simulink model "Exo_Origianl"  (R2023b)
settings: Solver=ode5  StartTime=0.0  StopTime=inf  FixedStep=dt  RelTol=1e-3  EnableMultiTasking=on
values from neighbouring files (symbols this model uses):
  A_0_a = 4.011    [Operator.m]
  A_0_h = 40.69    [Operator.m]
  A_0_k = 25.7    [Operator.m]
  A_1_a = 5.292    [Operator.m]
  A_1_h = 23.22    [Operator.m]
  A_1_k = -3.827    [Operator.m]
  A_2_a = -8.582    [Operator.m]
  A_2_h = -4.487    [Operator.m]
  A_2_k = -8.543    [Operator.m]
  A_3_a = -0.4755    [Operator.m]
  A_3_h = 0.3995    [Operator.m]
  A_3_k = 1.913    [Operator.m]
  A_4_a = 1.688    [Operator.m]
  A_4_k = 1.087    [Operator.m]
  A_5_a = -0.03504    [Operator.m]
  A_5_k = 2.054    [Operator.m]
  A_6_a = 1.298    [Operator.m]
  A_6_k = -0.3061    [Operator.m]
  amplitude = 0.8    [Operator.m]
  ankleStrategyInterval = 1.5    [Operator.m]
  B_1_a = 3.613    [Operator.m]
  B_1_h = -8.65    [Operator.m]
  B_1_k = -19.28    [Operator.m]
  B_2_a = -5.954    [Operator.m]
  B_2_h = 3.338    [Operator.m]
  B_2_k = 17.93    [Operator.m]
  B_3_a = 5.918    [Operator.m]
  B_3_h = 1.389    [Operator.m]
  B_3_k = 3.772    [Operator.m]
  B_4_a = -2.118    [Operator.m]
  B_4_k = 1.504    [Operator.m]
  B_5_a = 1.023    [Operator.m]
  B_5_k = 0.5838    [Operator.m]
  B_6_a = -0.7245    [Operator.m]
  B_6_k = -0.8958    [Operator.m]
  DCM_filter = 1 - dt/(dt+RC)    (= 0.926612305411)    [Operator.m]
  dt = 0.01    [Operator.m]
  frequency = 1.2    [Operator.m]
  gamma = fzero(eqn, 0.1)    [Operator.m]
  hipOffset = -17    [Operator.m]
  K_high = 0.5    [Operator.m]
  K_low = 0.5    [Operator.m]
  KD = 0.39    [Operator.m]
  Kp = 10    [Operator.m]
  l3 = userHeight*0.232    (= 15.776)    [Operator.m]
  l4 = userHeight*0.247    (= 16.796)    [Operator.m]
  l_c2 = ((0.29*34.66+0.63*6.07)/(6.07+34.66))/(0.52+0.19)*l2    (= 15.0425832454)    [Operator.m]
  l_c3 = 0.17/0.40*l3    (= 6.7048)    [Operator.m]
  l_c4 = ((0.19*3.52+0.43*1.05)/(3.52+1.05))/0.43*l4    (= 9.57536959951)    [Operator.m]
  l_foot = 11.25    [Operator.m]
  m2 = m2 + 2.2048*7.591    (= 119.8566368)    [Operator.m]
  m3 = m3 + 2.2048*1.715    (= 19.781232)    [Operator.m]
  m4 = userWeight*(0.0459+0.0169)    (= 10.048)    [Operator.m]
  m_Exo = 2.2048*1.647    (= 3.6313056)    [Operator.m]
  m_f = userWeight*0.0169    (= 2.704)    [Operator.m]
  maxTorque = 35    [Operator.m]
  P_t_ZMP_gain_Ankle = 0    [Operator.m]
  P_t_ZMP_gain_Hip = 0    [Operator.m]
  Phase_Left = 2+pi    (= 5.14159265359)    [Operator.m]
  Phase_Right = 2    [Operator.m]
  ramp = 2    [Operator.m]
  Strategy_filter = DCM_filter    (= 0.926612305411)    [Operator.m]
  strategySaturation = 10    [Operator.m]
  userHeight = 68    [Operator.m]
  userWeight = 160    [Operator.m]
undefined symbols (not defined in the file or in its folder): CAN_Device, DCMErrorPenalty, PEAK, Phase_Left_Knee_0, System, totalPowerPenalty
libraries: sldrtlib x35, simulink x16, rllib x1
(part 2 of 4)

== system Exo_Origianl/Subsystem1 ==
  In1 : Inport
  In2 : Inport  Port=2
  Trigger : TriggerPort  VariantControl=(inherit)  PortDimensions=1
  Constant{1..6} (6 alike) : Constant  Value=3
  Packet Output : sldrtlib/Packet Output  SampleTime=-1  MaxMissedTicks=100  ShowMissedTicks=off  YieldWhenWaiting=off  DrvName=PEAK-System/CAN_Device  DrvAddress=81  DrvOptions=[0 0 0 0 1000 0 0 1 5 2 1 3 1]  PacketSize=8  DataTypes={'uint8','uint8','uint8','uint8','uint8','uint8','uint8','uint8'}  ShowReady=off  ShowError=off  PacketID=2048e0 + (81)  ByteOrder=2  InitialValue=[]  FinalValue=[]
      settings: AttributesFormatString=PEAK-System\nCAN Device [81]
  wires:
  In2/1 -> Packet Output/2
  In1/1 -> Packet Output/1
  Constant1/1 -> Packet Output/7
  Constant6/1 -> Packet Output/8
  Constant2/1 -> Packet Output/3
  Constant3/1 -> Packet Output/4
  Constant4/1 -> Packet Output/5
  Constant5/1 -> Packet Output/6

== system Exo_Origianl/Subsystem10 ==
  In1 : Inport
  Trigger : TriggerPort  TriggerType=either  VariantControl=(inherit)  PortDimensions=1
  Constant{1..7} (7 alike) : Constant
  Packet Output : sldrtlib/Packet Output  SampleTime=-1  MaxMissedTicks=100  ShowMissedTicks=off  YieldWhenWaiting=off  DrvName=PEAK-System/CAN_Device  DrvAddress=81  DrvOptions=[0 0 0 0 1000 0 0 1 5 2 1 3 1]  PacketSize=8  DataTypes={'uint8','uint8','uint8','uint8','uint8','uint8','uint8','uint8'}  ShowReady=off  ShowError=off  PacketID=2048e0 + (85)  ByteOrder=2  InitialValue=[]  FinalValue=[]
      settings: AttributesFormatString=PEAK-System\nCAN Device [81]
  wires:
  Constant7/1 -> Packet Output/2
  In1/1 -> Packet Output/1
  Constant3/1 -> Packet Output/4
  Constant1/1 -> Packet Output/7
  Constant6/1 -> Packet Output/8
  Constant4/1 -> Packet Output/5
  Constant2/1 -> Packet Output/3
  Constant5/1 -> Packet Output/6

== system Exo_Origianl/Subsystem11 ==
  In1 : Inport
  In2 : Inport  Port=2
  Trigger : TriggerPort  VariantControl=(inherit)  PortDimensions=1
  Constant{1..6} (6 alike) : Constant
  Packet Output : sldrtlib/Packet Output  SampleTime=-1  MaxMissedTicks=100  ShowMissedTicks=off  YieldWhenWaiting=off  DrvName=PEAK-System/CAN_Device  DrvAddress=81  DrvOptions=[0 0 0 0 1000 0 0 1 5 2 1 3 1]  PacketSize=8  DataTypes={'uint8','uint8','uint8','uint8','uint8','uint8','uint8','uint8'}  ShowReady=off  ShowError=off  PacketID=2048e0 + (81)  ByteOrder=2  InitialValue=[]  FinalValue=[]
      settings: AttributesFormatString=PEAK-System\nCAN Device [81]
  wires:
  In2/1 -> Packet Output/2
  In1/1 -> Packet Output/1
  Constant4/1 -> Packet Output/5
  Constant6/1 -> Packet Output/8
  Constant1/1 -> Packet Output/7
  Constant3/1 -> Packet Output/4
  Constant5/1 -> Packet Output/6
  Constant2/1 -> Packet Output/3

== system Exo_Origianl/Subsystem12 ==
  Input : Inport
  Clock : Clock
  MATLAB Function : MATLAB Function  TreatAsAtomicUnit=on
  MATLAB Function1 : MATLAB Function  TreatAsAtomicUnit=on
  ramp : Constant  Value=ramp
  amplitude : Outport
  frequency : Outport  Port=2
  hipOffset : Outport  Port=3
  wires:
  MATLAB Function1/3(hipOffset) -> hipOffset/1
  MATLAB Function1/1(amplitude) -> amplitude/1
  Clock/1 -> MATLAB Function/1(clock)
  ramp/1 -> MATLAB Function1/3(ramp)
  MATLAB Function/1(Time) -> MATLAB Function1/1(clock)
  MATLAB Function1/2(frequency) -> frequency/1
  Input/1 -> MATLAB Function1/2(trigger), MATLAB Function/2(trigger)

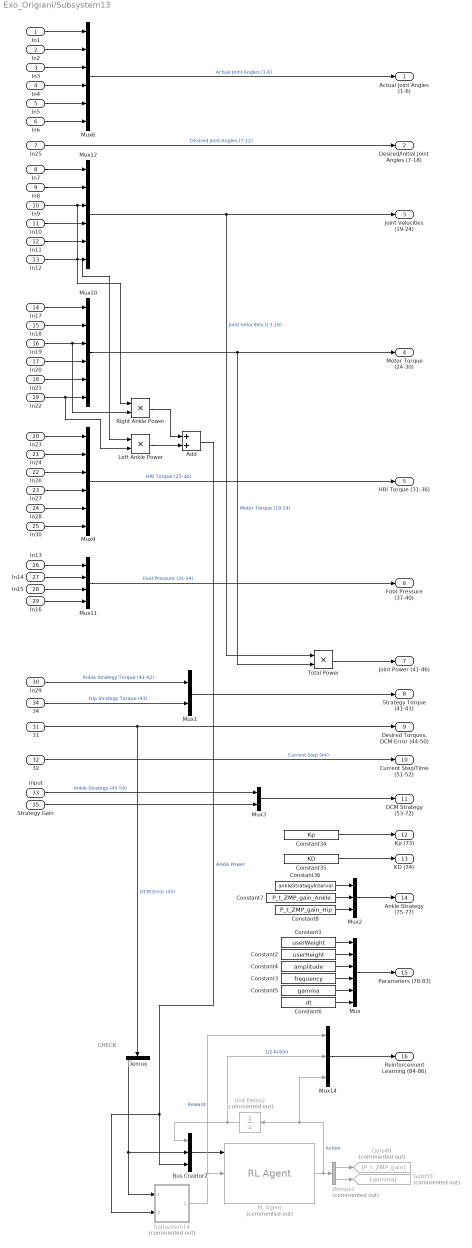
== system Exo_Origianl/Subsystem13 ==
  note: CHECK
  In1 : Inport
  In2 : Inport  Port=2
  In3 : Inport  Port=3
  In4 : Inport  Port=4
  In5 : Inport  Port=5
  In6 : Inport  Port=6
  In25 : Inport  Port=7
  In7 : Inport  Port=8
  In8 : Inport  Port=9
  In9 : Inport  Port=10
  In10 : Inport  Port=11
  In11 : Inport  Port=12
  In12 : Inport  Port=13
  In17 : Inport  Port=14
  In18 : Inport  Port=15
  In19 : Inport  Port=16
  In20 : Inport  Port=17
  In21 : Inport  Port=18
  In22 : Inport  Port=19
  In23 : Inport  Port=20
  In24 : Inport  Port=21
  In26 : Inport  Port=22
  In27 : Inport  Port=23
  In28 : Inport  Port=24
  In30 : Inport  Port=25
  In13 : Inport  Port=26
  In14 : Inport  Port=27
  In15 : Inport  Port=28
  In16 : Inport  Port=29
  In29 : Inport  Port=30
  31 : Inport  Port=31
  32 : Inport  Port=32
  Input : Inport  Port=33
  34 : Inport  Port=34
  Strategy Gain : Inport  Port=35
  Add : Sum
  Bus Creator2 : BusCreator  Inputs=3
  Constant1 : Constant  Value=userWeight
  Constant2 : Constant  Value=userHeight
  Constant3 : Constant  Value=frequency
  Constant34 : Constant  Value=Kp
  Constant35 : Constant  Value=KD
  Constant36 : Constant  Value=ankleStrategyInterval
  Constant4 : Constant  Value=amplitude
  Constant5 : Constant  Value=gamma
  Constant6 : Constant  Value=dt
  Constant7 : Constant  Value=P_t_ZMP_gain_Ankle
  Constant8 : Constant  Value=P_t_ZMP_gain_Hip
  Demux : Demux  Outputs=7
  Demux1 : Demux  Commented=on  Outputs=2
  Goto49 : Goto  Commented=on  GotoTag=P_t_ZMP_gain
  Goto50 : Goto  Commented=on  GotoTag=gamma
  Left Ankle Power : Product
  Mux{,6,9..10,12} (5 alike) : Mux  Inputs=6
  Mux1 : Mux  Inputs=2
  Mux11 : Mux
  Mux14 : Mux  Inputs=3
  Mux2 : Mux  Inputs=3
  Mux3 : Mux  Inputs=2
  RL Agent : rllib/RL Agent  Commented=on  Agent=agent  ExternalActionAsInput=off  ProvideLastAction=off  ProvideCumRwd=off  TreatAsDirectFeedthrough=on  UseStrictObservationDataTypes=off
  Right Ankle Power : Product
  Subsystem14 : Subsystem  Commented=on
  Total Power : Product
  Unit Delay2 : UnitDelay  Commented=on  SampleTime=-1  HasFrameUpgradeWarning=on
  Actual Joint Angles (1-6) : Outport
  Desired/Initial Joint Angles (7-18) : Outport  Port=2
  Joint Velocities (19-24) : Outport  Port=3
  Motor Torque (24-30) : Outport  Port=4
  HRI Torque (31-36) : Outport  Port=5
  Foot Pressure (37-40) : Outport  Port=6
  Joint Power (41-46) : Outport  Port=7
  Strategy Torque (41-43) : Outport  Port=8
  "Desired Torques, DCM Error (44-50)" : Outport  Port=9
  Current Step/Time (51-52) : Outport  Port=10
  DCM Strategy (53-72) : Outport  Port=11
  Kp (73) : Outport  Port=12
  KD (74) : Outport  Port=13
  Ankle Strategy (75-77) : Outport  Port=14
  Parameters (78-83) : Outport  Port=15
  Reinforcement Learning (84-86) : Outport  Port=16
  wires:
  Mux14/1 -> Reinforcement Learning (84-86)/1
  In3/1 -> Mux6/3
  Mux6/1 -> Actual Joint Angles (1-6)/1  "Actual Joint Angles (1-6)"
  In20/1 -> Mux10/4
  In15/1 -> Mux11/3
  Demux1/2 -> Goto50/1
  In13/1 -> Mux11/1
  In21/1 -> Mux10/5
  In24/1 -> Mux9/2
  In23/1 -> Mux9/1
  In18/1 -> Mux10/2
  31/1 -> "Desired Torques, DCM Error (44-50)"/1, Demux/1  "DCM Error (43)"
  In7/1 -> Mux12/1
  In2/1 -> Mux6/2
  Mux9/1 -> HRI Torque (31-36)/1  "HRI Torque (25-30)"
  Right Ankle Power/1 -> Add/1
  In6/1 -> Mux6/6
  In30/1 -> Mux9/6
  In1/1 -> Mux6/1
  In8/1 -> Mux12/2
  In22/1 -> Mux10/6, Left Ankle Power/2
  In12/1 -> Mux12/6, Left Ankle Power/1
  In11/1 -> Mux12/5
  Bus Creator2/1 -> RL Agent/1
  In5/1 -> Mux6/5
  In28/1 -> Mux9/5
  Add/1 -> Subsystem14/2(Power), Bus Creator2/3  "Ankle Power"
  Mux11/1 -> Foot Pressure (37-40)/1  "Foot Pressure (31-34)"
  In27/1 -> Mux9/4
  In10/1 -> Mux12/4
  In26/1 -> Mux9/3
  In16/1 -> Mux11/4
  Mux12/1 -> Joint Velocities (19-24)/1, Total Power/1  "Joint Velocities (13-18)"
  In17/1 -> Mux10/1
  In4/1 -> Mux6/4
  In9/1 -> Mux12/3, Right Ankle Power/1
  Mux10/1 -> Motor Torque (24-30)/1, Total Power/2  "Motor Torque (19-24)"
  In19/1 -> Mux10/3, Right Ankle Power/2
  RL Agent/1 -> Unit Delay2/1, Mux14/3, Demux1/1  "Action"
  Demux1/1 -> Goto49/1
  Total Power/1 -> Joint Power (41-46)/1
  In14/1 -> Mux11/2
  Left Ankle Power/1 -> Add/2
  Unit Delay2/1 -> Mux14/2, Bus Creator2/1  "1/z Action"
  Subsystem14/1(Reward) -> RL Agent/2, Mux14/1  "Reward"
  In25/1 -> Desired/Initial Joint Angles (7-18)/1  "Desired Joint Angles (7-12)"
  Constant34/1 -> Kp (73)/1
  Constant35/1 -> KD (74)/1
  Mux2/1 -> Ankle Strategy (75-77)/1
  In29/1 -> Mux1/1  "Ankle Strategy Torque (41-42)"
  32/1 -> Current Step/Time (51-52)/1  "Current Step (44)"
  Input/1 -> Mux3/1  "Ankle Strategy (45-54)"
  Demux/1 -> Bus Creator2/2, Subsystem14/1(DCM Error)
  Constant1/1 -> Mux/1
  Constant2/1 -> Mux/2
  Constant4/1 -> Mux/3
  Constant3/1 -> Mux/4
  Constant5/1 -> Mux/5
  Constant6/1 -> Mux/6
  Mux/1 -> Parameters (78-83)/1
  34/1 -> Mux1/2  "Hip Strategy Torque (43)"
  Mux1/1 -> Strategy Torque (41-43)/1
  Constant36/1 -> Mux2/1
  Constant7/1 -> Mux2/2
  Constant8/1 -> Mux2/3
  Mux3/1 -> DCM Strategy (53-72)/1
  Strategy Gain/1 -> Mux3/2

== system Exo_Origianl/Subsystem15 ==
  Input : Inport
  Input1 : Inport  Port=2
  Input2 : Inport  Port=3
  AND : Logic  Inputs=3  IconShape=distinctive  AllPortsSameDT=off  OutDataTypeStr=boolean
  Cast To Double1 : DataTypeConversion  OutDataTypeStr=double  SaturateOnIntegerOverflow=off  RndMeth=Floor
  If2 : If
  Subsystem14 : Subsystem
  Trigger : Outport
  wires:
  Cast To Double1/1 -> If2/1
  AND/1 -> Cast To Double1/1
  If2/1 -> Trigger/1
  Input/1 -> AND/1
  Subsystem14/1(Out1) -> AND/2
  Input1/1 -> Subsystem14/1(Input)
  Input2/1 -> AND/3

== system Exo_Origianl/Subsystem2 ==
  In1 : Inport
  In2 : Inport  Port=2
  Trigger : TriggerPort  VariantControl=(inherit)  PortDimensions=1
  Constant{1..6} (6 alike) : Constant
  Packet Output : sldrtlib/Packet Output  SampleTime=-1  MaxMissedTicks=100  ShowMissedTicks=off  YieldWhenWaiting=off  DrvName=PEAK-System/CAN_Device  DrvAddress=81  DrvOptions=[0 0 0 0 1000 0 0 1 5 2 1 3 1]  PacketSize=8  DataTypes={'uint8','uint8','uint8','uint8','uint8','uint8','uint8','uint8'}  ShowReady=off  ShowError=off  PacketID=2048e0 + (81)  ByteOrder=2  InitialValue=[]  FinalValue=[]
      settings: AttributesFormatString=PEAK-System\nCAN Device [81]
  wires:
  In1/1 -> Packet Output/1
  In2/1 -> Packet Output/2
  Constant1/1 -> Packet Output/7
  Constant6/1 -> Packet Output/8
  Constant2/1 -> Packet Output/3
  Constant3/1 -> Packet Output/4
  Constant4/1 -> Packet Output/5
  Constant5/1 -> Packet Output/6

== system Exo_Origianl/Subsystem3 ==
  In1 : Inport
  In2 : Inport  Port=2
  Trigger : TriggerPort  VariantControl=(inherit)  PortDimensions=1
  Constant{1..6} (6 alike) : Constant
  Packet Output : sldrtlib/Packet Output  SampleTime=-1  MaxMissedTicks=100  ShowMissedTicks=off  YieldWhenWaiting=off  DrvName=PEAK-System/CAN_Device  DrvAddress=81  DrvOptions=[0 0 0 0 1000 0 0 1 5 2 1 3 1]  PacketSize=8  DataTypes={'uint8','uint8','uint8','uint8','uint8','uint8','uint8','uint8'}  ShowReady=off  ShowError=off  PacketID=2048e0 + (81)  ByteOrder=2  InitialValue=[]  FinalValue=[]
      settings: AttributesFormatString=PEAK-System\nCAN Device [81]
  wires:
  In2/1 -> Packet Output/2
  In1/1 -> Packet Output/1
  Constant3/1 -> Packet Output/4
  Constant1/1 -> Packet Output/7
  Constant6/1 -> Packet Output/8
  Constant4/1 -> Packet Output/5
  Constant2/1 -> Packet Output/3
  Constant5/1 -> Packet Output/6

== system Exo_Origianl/Subsystem4 ==
  In1 : Inport
  In2 : Inport  Port=2
  Trigger : TriggerPort  VariantControl=(inherit)  PortDimensions=1
  Constant{1..6} (6 alike) : Constant
  Packet Output : sldrtlib/Packet Output  SampleTime=-1  MaxMissedTicks=100  ShowMissedTicks=off  YieldWhenWaiting=off  DrvName=PEAK-System/CAN_Device  DrvAddress=81  DrvOptions=[0 0 0 0 1000 0 0 1 5 2 1 3 1]  PacketSize=8  DataTypes={'uint8','uint8','uint8','uint8','uint8','uint8','uint8','uint8'}  ShowReady=off  ShowError=off  PacketID=2048e0 + (81)  ByteOrder=2  InitialValue=[]  FinalValue=[]
      settings: AttributesFormatString=PEAK-System\nCAN Device [81]
  wires:
  In1/1 -> Packet Output/1
  In2/1 -> Packet Output/2
  Constant3/1 -> Packet Output/4
  Constant1/1 -> Packet Output/7
  Constant6/1 -> Packet Output/8
  Constant4/1 -> Packet Output/5
  Constant2/1 -> Packet Output/3
  Constant5/1 -> Packet Output/6

== system Exo_Origianl/Subsystem5 ==
  In1 : Inport
  In2 : Inport  Port=2
  Trigger : TriggerPort  VariantControl=(inherit)  PortDimensions=1
  Constant{1..6} (6 alike) : Constant
  Packet Output : sldrtlib/Packet Output  SampleTime=-1  MaxMissedTicks=100  ShowMissedTicks=off  YieldWhenWaiting=off  DrvName=PEAK-System/CAN_Device  DrvAddress=81  DrvOptions=[0 0 0 0 1000 0 0 1 5 2 1 3 1]  PacketSize=8  DataTypes={'uint8','uint8','uint8','uint8','uint8','uint8','uint8','uint8'}  ShowReady=off  ShowError=off  PacketID=2048e0 + (81)  ByteOrder=2  InitialValue=[]  FinalValue=[]
      settings: AttributesFormatString=PEAK-System\nCAN Device [81]
  wires:
  In2/1 -> Packet Output/2
  In1/1 -> Packet Output/1
  Constant3/1 -> Packet Output/4
  Constant1/1 -> Packet Output/7
  Constant6/1 -> Packet Output/8
  Constant4/1 -> Packet Output/5
  Constant2/1 -> Packet Output/3
  Constant5/1 -> Packet Output/6

== system Exo_Origianl/Subsystem6 ==
  In1 : Inport
  In2 : Inport  Port=2
  In3 : Inport  Port=3
  Trigger : TriggerPort  VariantControl=(inherit)  PortDimensions=1
  Constant{1,3..6} (5 alike) : Constant
  Packet Output : sldrtlib/Packet Output  SampleTime=-1  MaxMissedTicks=100  ShowMissedTicks=off  YieldWhenWaiting=off  DrvName=PEAK-System/CAN_Device  DrvAddress=81  DrvOptions=[0 0 0 0 1000 0 0 1 5 2 1 3 1]  PacketSize=8  DataTypes={'uint8','uint8','uint8','uint8','uint8','uint8','uint8','uint8'}  ShowReady=off  ShowError=off  PacketID=2048e0 + (81)  ByteOrder=2  InitialValue=[]  FinalValue=[]
      settings: AttributesFormatString=PEAK-System\nCAN Device [81]
  wires:
  In1/1 -> Packet Output/1
  Constant4/1 -> Packet Output/5
  Constant6/1 -> Packet Output/8
  Constant1/1 -> Packet Output/7
  Constant3/1 -> Packet Output/4
  Constant5/1 -> Packet Output/6
  In2/1 -> Packet Output/2
  In3/1 -> Packet Output/3

== system Exo_Origianl/Subsystem7 ==
  In1 : Inport
  In2 : Inport  Port=2
  Trigger : TriggerPort  VariantControl=(inherit)  PortDimensions=1
  Constant{1..6} (6 alike) : Constant
  Packet Output : sldrtlib/Packet Output  SampleTime=-1  MaxMissedTicks=100  ShowMissedTicks=off  YieldWhenWaiting=off  DrvName=PEAK-System/CAN_Device  DrvAddress=81  DrvOptions=[0 0 0 0 1000 0 0 1 5 2 1 3 1]  PacketSize=8  DataTypes={'uint8','uint8','uint8','uint8','uint8','uint8','uint8','uint8'}  ShowReady=off  ShowError=off  PacketID=2048e0 + (81)  ByteOrder=2  InitialValue=[]  FinalValue=[]
      settings: AttributesFormatString=PEAK-System\nCAN Device [81]
  wires:
  In2/1 -> Packet Output/2
  In1/1 -> Packet Output/1
  Constant4/1 -> Packet Output/5
  Constant6/1 -> Packet Output/8
  Constant1/1 -> Packet Output/7
  Constant3/1 -> Packet Output/4
  Constant5/1 -> Packet Output/6
  Constant2/1 -> Packet Output/3

== system Exo_Origianl/Subsystem8 ==
  In1 : Inport
  In2 : Inport  Port=2
  Trigger : TriggerPort  VariantControl=(inherit)  PortDimensions=1
  Constant{1..6} (6 alike) : Constant  Value=0
  Packet Output : sldrtlib/Packet Output  SampleTime=-1  MaxMissedTicks=100  ShowMissedTicks=off  YieldWhenWaiting=off  DrvName=PEAK-System/CAN_Device  DrvAddress=81  DrvOptions=[0 0 0 0 1000 0 0 1 5 2 1 3 1]  PacketSize=8  DataTypes={'uint8','uint8','uint8','uint8','uint8','uint8','uint8','uint8'}  ShowReady=off  ShowError=off  PacketID=2048e0 + (81)  ByteOrder=2  InitialValue=[]  FinalValue=[]
      settings: AttributesFormatString=PEAK-System\nCAN Device [81]
  wires:
  In1/1 -> Packet Output/1
  In2/1 -> Packet Output/2
  Constant3/1 -> Packet Output/4
  Constant5/1 -> Packet Output/6
  Constant4/1 -> Packet Output/5
  Constant6/1 -> Packet Output/8
  Constant1/1 -> Packet Output/7
  Constant2/1 -> Packet Output/3

== system Exo_Origianl/Subsystem9 ==
  In1 : Inport
  In2 : Inport  Port=2
  Trigger : TriggerPort  VariantControl=(inherit)  PortDimensions=1
  Constant{1..6} (6 alike) : Constant  Value=0
  Packet Output : sldrtlib/Packet Output  SampleTime=-1  MaxMissedTicks=100  ShowMissedTicks=off  YieldWhenWaiting=off  DrvName=PEAK-System/CAN_Device  DrvAddress=81  DrvOptions=[0 0 0 0 1000 0 0 1 5 2 1 3 1]  PacketSize=8  DataTypes={'uint8','uint8','uint8','uint8','uint8','uint8','uint8','uint8'}  ShowReady=off  ShowError=off  PacketID=2048e0 + (81)  ByteOrder=2  InitialValue=[]  FinalValue=[]
      settings: AttributesFormatString=PEAK-System\nCAN Device [81]
  wires:
  In2/1 -> Packet Output/2
  In1/1 -> Packet Output/1
  Constant3/1 -> Packet Output/4
  Constant5/1 -> Packet Output/6
  Constant4/1 -> Packet Output/5
  Constant6/1 -> Packet Output/8
  Constant1/1 -> Packet Output/7
  Constant2/1 -> Packet Output/3

== system Exo_Origianl/Up and Down Assistance % Left ==
  Constant2 : Constant  Value=0
  Constant9 : Constant  Value=0
  Detect Change : simulink/Logic and Bit Operations/Detect Change  vinit=0  OutDataTypeStr=uint8
  Subsystem : Subsystem
  Out1 : Outport
  Out2 : Outport  Port=2
  Out3 : Outport  Port=3
  wires:
  Subsystem/1(Out1) -> Out1/1
  Constant9/1 -> Subsystem/1(In1)
  Subsystem/2(Out2) -> Detect Change/1, Out2/1
  Detect Change/1 -> Out3/1
  Constant2/1 -> Subsystem/2(In2)

== system Exo_Origianl/Up and Down Assistance % Right ==
  Constant2 : Constant  Value=0
  Constant9 : Constant  Value=0
  Detect Change : simulink/Logic and Bit Operations/Detect Change  vinit=0  OutDataTypeStr=uint8
  Subsystem : Subsystem
  Out1 : Outport
  Out2 : Outport  Port=2
  Out3 : Outport  Port=3
  wires:
  Subsystem/1(Out1) -> Out1/1
  Constant2/1 -> Subsystem/2(In2)
  Constant9/1 -> Subsystem/1(In1)
  Subsystem/2(Out2) -> Detect Change/1, Out2/1
  Detect Change/1 -> Out3/1

== system Exo_Origianl/Up and Down Speed ==
  Constant3 : Constant  Value=0
  Constant9 : Constant  Value=0
  Detect Change : simulink/Logic and Bit Operations/Detect Change  vinit=0  OutDataTypeStr=uint8
  Subsystem : Subsystem
  Out1 : Outport
  Out2 : Outport  Port=2
  wires:
  Constant9/1 -> Subsystem/2(In2)
  Subsystem/1(Out1) -> Detect Change/1, Out1/1
  Constant3/1 -> Subsystem/1(In1)
  Detect Change/1 -> Out2/1

== system Exo_Origianl/Exo State/If Action Subsystem ==
  Action Port : ActionPort  ActionPortLabel=if(u1 == 1)
  Data Type Conversion{6..11} (6 alike) : DataTypeConversion  OutDataTypeStr=double  SaturateOnIntegerOverflow=off  RndMeth=Floor
  Packet Input1 : sldrtlib/Packet Input  SampleTime=-1  MaxMissedTicks=10  ShowMissedTicks=off  YieldWhenWaiting=off  DrvName=PEAK-System/CAN_Device  DrvAddress=81  DrvOptions=[0 0 0 0 1000 0 0 1 5 2 1 3 1]  PacketSize=6  DataTypes={'uint8','uint8','uint8','uint8','uint8','uint8'}  ShowReady=off  ShowError=off  PacketID=2048e0 + (150)  ByteOrder=1  ShowTimestamp=off
      settings: AttributesFormatString=PEAK-System\nCAN Device [81]
  Out7 : Outport
  Out8 : Outport  Port=2
  Out9 : Outport  Port=3
  Out10 : Outport  Port=4
  Out11 : Outport  Port=5
  Out12 : Outport  Port=6
  wires:
  Data Type Conversion10/1 -> Out11/1
  Packet Input1/6 -> Data Type Conversion11/1
  Data Type Conversion11/1 -> Out12/1
  Packet Input1/5 -> Data Type Conversion10/1
  Data Type Conversion7/1 -> Out8/1
  Packet Input1/4 -> Data Type Conversion9/1
  Data Type Conversion6/1 -> Out7/1
  Packet Input1/2 -> Data Type Conversion7/1
  Data Type Conversion8/1 -> Out9/1
  Packet Input1/1 -> Data Type Conversion6/1
  Data Type Conversion9/1 -> Out10/1
  Packet Input1/3 -> Data Type Conversion8/1

== system Exo_Origianl/Exo State/If Action Subsystem1 ==
  Action Port : ActionPort  ActionPortLabel=else
  Data Type Conversion{6..11} (6 alike) : DataTypeConversion  OutDataTypeStr=double  SaturateOnIntegerOverflow=off  RndMeth=Floor
  Packet Input1 : sldrtlib/Packet Input  SampleTime=-1  MaxMissedTicks=10  ShowMissedTicks=off  YieldWhenWaiting=off  DrvName=PEAK-System/CAN_Device  DrvAddress=81  DrvOptions=[0 0 0 0 1000 0 0 1 5 2 1 3 1]  PacketSize=6  DataTypes={'uint8','uint8','uint8','uint8','uint8','uint8'}  ShowReady=off  ShowError=off  PacketID=2048e0 + (59)  ByteOrder=1  ShowTimestamp=off
      settings: AttributesFormatString=PEAK-System\nCAN Device [81]
  Out1 : Outport
  Out2 : Outport  Port=2
  Out3 : Outport  Port=3
  Out4 : Outport  Port=4
  Out5 : Outport  Port=5
  Out6 : Outport  Port=6
  wires:
  Packet Input1/3 -> Data Type Conversion8/1
  Data Type Conversion9/1 -> Out4/1
  Data Type Conversion6/1 -> Out1/1
  Packet Input1/2 -> Data Type Conversion7/1
  Packet Input1/1 -> Data Type Conversion6/1
  Packet Input1/4 -> Data Type Conversion9/1
  Packet Input1/5 -> Data Type Conversion10/1
  Data Type Conversion8/1 -> Out3/1
  Data Type Conversion10/1 -> Out5/1
  Data Type Conversion7/1 -> Out2/1
  Packet Input1/6 -> Data Type Conversion11/1
  Data Type Conversion11/1 -> Out6/1

== system Exo_Origianl/Exo State 2/If Action Subsystem ==
  Action Port : ActionPort  ActionPortLabel=if(u1 == 1)
  Constant : Constant  Value=0
  Out7 : Outport
  Out8 : Outport  Port=2
  Out9 : Outport  Port=3
  Out10 : Outport  Port=4
  Out11 : Outport  Port=5
  Out12 : Outport  Port=6
  wires:
  Constant/1 -> Out7/1, Out8/1, Out9/1, Out12/1, Out11/1, Out10/1

== system Exo_Origianl/Exo State 2/If Action Subsystem1 ==
  Action Port : ActionPort  ActionPortLabel=else
  Data Type Conversion{6..11} (6 alike) : DataTypeConversion  OutDataTypeStr=double  SaturateOnIntegerOverflow=off  RndMeth=Floor
  Packet Input1 : sldrtlib/Packet Input  SampleTime=-1  MaxMissedTicks=10  ShowMissedTicks=off  YieldWhenWaiting=off  DrvName=PEAK-System/CAN_Device  DrvAddress=81  DrvOptions=[0 0 0 0 1000 0 0 1 5 2 1 3 1]  PacketSize=6  DataTypes={'uint8','uint8','uint8','uint8','uint8','uint8'}  ShowReady=off  ShowError=off  PacketID=2048e0 + (60)  ByteOrder=1  ShowTimestamp=off
      settings: AttributesFormatString=PEAK-System\nCAN Device [81]
  Out1 : Outport
  Out2 : Outport  Port=2
  Out3 : Outport  Port=3
  Out4 : Outport  Port=4
  Out5 : Outport  Port=5
  Out6 : Outport  Port=6
  wires:
  Packet Input1/3 -> Data Type Conversion8/1
  Data Type Conversion9/1 -> Out4/1
  Data Type Conversion6/1 -> Out1/1
  Packet Input1/2 -> Data Type Conversion7/1
  Packet Input1/1 -> Data Type Conversion6/1
  Packet Input1/4 -> Data Type Conversion9/1
  Packet Input1/5 -> Data Type Conversion10/1
  Data Type Conversion8/1 -> Out3/1
  Data Type Conversion10/1 -> Out5/1
  Data Type Conversion7/1 -> Out2/1
  Packet Input1/6 -> Data Type Conversion11/1
  Data Type Conversion11/1 -> Out6/1

== system Exo_Origianl/Exo States Messages/Switch Case Action Subsystem ==
  Action Port : ActionPort  ActionPortLabel=case [ 1 ]:
  String Constant1 : StringConstant  String="\"Walking at the desired speed 1\""
  Out1 : Outport
  wires:
  String Constant1/1 -> Out1/1

== system Exo_Origianl/Exo States Messages/Switch Case Action Subsystem1 ==
  Action Port : ActionPort  ActionPortLabel=case [ 2 ]:
  String Constant1 : StringConstant  String="\"Walking at the desired speed 2\""
  Out1 : Outport
  wires:
  String Constant1/1 -> Out1/1

== system Exo_Origianl/Exo States Messages/Switch Case Action Subsystem10 ==
  Action Port : ActionPort  ActionPortLabel=case [ 0 ]:
  String Constant : StringConstant  String="\"Standing\""
  Out1 : Outport
  wires:
  String Constant/1 -> Out1/1

== system Exo_Origianl/Exo States Messages/Switch Case Action Subsystem11 ==
  Action Port : ActionPort  ActionPortLabel=case [ 11 ]:
  String Constant11 : StringConstant  String="\"Joints in release mode\""
  Out1 : Outport
  wires:
  String Constant11/1 -> Out1/1

== system Exo_Origianl/Exo States Messages/Switch Case Action Subsystem12 ==
  Action Port : ActionPort  ActionPortLabel=case [ 12 ]:
  String Constant12 : StringConstant  String="\"Joints in free mode\""
  Out1 : Outport
  wires:
  String Constant12/1 -> Out1/1

== system Exo_Origianl/Exo States Messages/Switch Case Action Subsystem13 ==
  Action Port : ActionPort  ActionPortLabel=case [ 13 ]:
  String Constant13 : StringConstant  String="\"stop Walking\""
  Out1 : Outport
  wires:
  String Constant13/1 -> Out1/1

== system Exo_Origianl/Exo States Messages/Switch Case Action Subsystem14 ==
  Action Port : ActionPort  ActionPortLabel=case [ 14 ]:
  String Constant14 : StringConstant  String="\"Standing\""
  Out1 : Outport
  wires:
  String Constant14/1 -> Out1/1

== system Exo_Origianl/Exo States Messages/Switch Case Action Subsystem15 ==
  Action Port : ActionPort  ActionPortLabel=case [ 15 ]:
  String Constant15 : StringConstant  String="\"Sitting\""
  Out1 : Outport
  wires:
  String Constant15/1 -> Out1/1

== system Exo_Origianl/Exo States Messages/Switch Case Action Subsystem16 ==
  Action Port : ActionPort  ActionPortLabel=case [ 16 ]:
  String Constant16 : StringConstant  String="\"Seated\""
  Out1 : Outport
  wires:
  String Constant16/1 -> Out1/1

== system Exo_Origianl/Exo States Messages/Switch Case Action Subsystem17 ==
  Action Port : ActionPort  ActionPortLabel=case [ 17 ]:
  String Constant17 : StringConstant  String="\"Stepping with left leg. Only in step by step mode\""
  Out1 : Outport
  wires:
  String Constant17/1 -> Out1/1

== system Exo_Origianl/Exo States Messages/Switch Case Action Subsystem18 ==
  Action Port : ActionPort  ActionPortLabel=case [ 18 ]:
  String Constant18 : StringConstant  String="\"Stepping with left right. Only in step by step mode\""
  Out1 : Outport
  wires:
  String Constant18/1 -> Out1/1

== system Exo_Origianl/Exo States Messages/Switch Case Action Subsystem19 ==
  Action Port : ActionPort  ActionPortLabel=case [ 19 ]:
  String Constant19 : StringConstant  String="\"Joints locked in current position\""
  Out1 : Outport
  wires:
  String Constant19/1 -> Out1/1

== system Exo_Origianl/Exo States Messages/Switch Case Action Subsystem2 ==
  Action Port : ActionPort  ActionPortLabel=case [ 3 ]:
  String Constant1 : StringConstant  String="\"Walking at the desired speed 3\""
  Out1 : Outport
  wires:
  String Constant1/1 -> Out1/1

== system Exo_Origianl/Exo States Messages/Switch Case Action Subsystem20 ==
  Action Port : ActionPort  ActionPortLabel=case [ 26 ]:
  String Constant26 : StringConstant  String="\"Malfunction in left ankle\""
  Out1 : Outport
  wires:
  String Constant26/1 -> Out1/1

== system Exo_Origianl/Exo States Messages/Switch Case Action Subsystem22 ==
  Action Port : ActionPort  ActionPortLabel=case [ 21 ]:
  String Constant21 : StringConstant  String="\"Malfunction in right hip\""
  Out1 : Outport
  wires:
  String Constant21/1 -> Out1/1

== system Exo_Origianl/Exo States Messages/Switch Case Action Subsystem23 ==
  Action Port : ActionPort  ActionPortLabel=case [ 22 ]:
  String Constant22 : StringConstant  String="\"Malfunction in right knee\""
  Out1 : Outport
  wires:
  String Constant22/1 -> Out1/1

== system Exo_Origianl/Exo States Messages/Switch Case Action Subsystem24 ==
  Action Port : ActionPort  ActionPortLabel=case [ 23 ]:
  String Constant23 : StringConstant  String="\"Malfunction in right ankle\""
  Out1 : Outport
  wires:
  String Constant23/1 -> Out1/1

== system Exo_Origianl/Exo States Messages/Switch Case Action Subsystem25 ==
  Action Port : ActionPort  ActionPortLabel=case [ 24 ]:
  String Constant24 : StringConstant  String="\"Malfunction in left hip\""
  Out1 : Outport
  wires:
  String Constant24/1 -> Out1/1

== system Exo_Origianl/Exo States Messages/Switch Case Action Subsystem26 ==
  Action Port : ActionPort  ActionPortLabel=case [ 25 ]:
  String Constant25 : StringConstant  String="\"Malfunction in left knee\""
  Out1 : Outport
  wires:
  String Constant25/1 -> Out1/1

== system Exo_Origianl/Exo States Messages/Switch Case Action Subsystem3 ==
  Action Port : ActionPort  ActionPortLabel=case [ 4 ]:
  String Constant1 : StringConstant  String="\"Walking at the desired speed 4\""
  Out1 : Outport
  wires:
  String Constant1/1 -> Out1/1

== system Exo_Origianl/Exo States Messages/Switch Case Action Subsystem4 ==
  Action Port : ActionPort  ActionPortLabel=case [ 5 ]:
  String Constant1 : StringConstant  String="\"Walking at the desired speed 5\""
  Out1 : Outport
  wires:
  String Constant1/1 -> Out1/1

== system Exo_Origianl/Exo States Messages/Switch Case Action Subsystem5 ==
  Action Port : ActionPort  ActionPortLabel=case [ 6 ]:
  String Constant1 : StringConstant  String="\"Walking at the desired speed 6\""
  Out1 : Outport
  wires:
  String Constant1/1 -> Out1/1

== system Exo_Origianl/Exo States Messages/Switch Case Action Subsystem6 ==
  Action Port : ActionPort  ActionPortLabel=case [ 7 ]:
  String Constant1 : StringConstant  String="\"Walking at the desired speed 7\""
  Out1 : Outport
  wires:
  String Constant1/1 -> Out1/1

== system Exo_Origianl/Exo States Messages/Switch Case Action Subsystem7 ==
  Action Port : ActionPort  ActionPortLabel=case [ 8 ]:
  String Constant1 : StringConstant  String="\"Walking at the desired speed 8\""
  Out1 : Outport
  wires:
  String Constant1/1 -> Out1/1

== system Exo_Origianl/Exo States Messages/Switch Case Action Subsystem8 ==
  Action Port : ActionPort  ActionPortLabel=case [ 9 ]:
  String Constant1 : StringConstant  String="\"Walking at the desired speed 9\""
  Out1 : Outport
  wires:
  String Constant1/1 -> Out1/1

== system Exo_Origianl/Exo States Messages/Switch Case Action Subsystem9 ==
  Action Port : ActionPort  ActionPortLabel=case [ 10 ]:
  String Constant1 : StringConstant  String="\"Walking at the desired speed 10\""
  Out1 : Outport
  wires:
  String Constant1/1 -> Out1/1

== system Exo_Origianl/Foot Sensor//Battery//Trigger/If Action Subsystem ==
  Action Port : ActionPort  ActionPortLabel=if(u1 == 1)
  Data Type Conversion{6..11} (6 alike) : DataTypeConversion  OutDataTypeStr=double  SaturateOnIntegerOverflow=off  RndMeth=Floor
  Packet Input1 : sldrtlib/Packet Input  SampleTime=-1  MaxMissedTicks=10  ShowMissedTicks=off  YieldWhenWaiting=off  DrvName=PEAK-System/CAN_Device  DrvAddress=81  DrvOptions=[0 0 0 0 1000 0 0 1 5 2 1 3 1]  PacketSize=6  DataTypes={'uint8','uint8','uint8','uint8','uint8','uint8'}  ShowReady=off  ShowError=off  PacketID=2048e0 + (130)  ByteOrder=1  ShowTimestamp=off
      settings: AttributesFormatString=PEAK-System\nCAN Device [81]
  Out7 : Outport
  Out8 : Outport  Port=2
  Out9 : Outport  Port=3
  Out10 : Outport  Port=4
  Out11 : Outport  Port=5
  Out12 : Outport  Port=6
  wires:
  Data Type Conversion10/1 -> Out11/1
  Packet Input1/6 -> Data Type Conversion11/1
  Data Type Conversion11/1 -> Out12/1
  Packet Input1/5 -> Data Type Conversion10/1
  Data Type Conversion7/1 -> Out8/1
  Packet Input1/4 -> Data Type Conversion9/1
  Data Type Conversion6/1 -> Out7/1
  Packet Input1/2 -> Data Type Conversion7/1
  Data Type Conversion8/1 -> Out9/1
  Packet Input1/1 -> Data Type Conversion6/1
  Data Type Conversion9/1 -> Out10/1
  Packet Input1/3 -> Data Type Conversion8/1

== system Exo_Origianl/Foot Sensor//Battery//Trigger/If Action Subsystem1 ==
  Action Port : ActionPort  ActionPortLabel=else
  Data Type Conversion{6..11} (6 alike) : DataTypeConversion  OutDataTypeStr=double  SaturateOnIntegerOverflow=off  RndMeth=Floor
  Packet Input1 : sldrtlib/Packet Input  SampleTime=-1  MaxMissedTicks=10  ShowMissedTicks=off  YieldWhenWaiting=off  DrvName=PEAK-System/CAN_Device  DrvAddress=81  DrvOptions=[0 0 0 0 1000 0 0 1 5 2 1 3 1]  PacketSize=6  DataTypes={'uint8','uint8','uint8','uint8','uint8','uint8'}  ShowReady=off  ShowError=off  PacketID=2048e0 + (58)  ByteOrder=1  ShowTimestamp=off
      settings: AttributesFormatString=PEAK-System\nCAN Device [81]
  Out1 : Outport
  Out2 : Outport  Port=2
  Out3 : Outport  Port=3
  Out4 : Outport  Port=4
  Out5 : Outport  Port=5
  Out6 : Outport  Port=6
  wires:
  Packet Input1/3 -> Data Type Conversion8/1
  Data Type Conversion9/1 -> Out4/1
  Data Type Conversion6/1 -> Out1/1
  Packet Input1/2 -> Data Type Conversion7/1
  Packet Input1/1 -> Data Type Conversion6/1
  Packet Input1/4 -> Data Type Conversion9/1
  Packet Input1/5 -> Data Type Conversion10/1
  Data Type Conversion8/1 -> Out3/1
  Data Type Conversion10/1 -> Out5/1
  Data Type Conversion7/1 -> Out2/1
  Packet Input1/6 -> Data Type Conversion11/1
  Data Type Conversion11/1 -> Out6/1

== system Exo_Origianl/If Action Subsystem3/Fourier Series ==
  A : Inport
  W : Inport  Port=2
  Offset : Inport  Port=3
  Left Ankle : Subsystem
  Left Hip : Subsystem
  Left Knee : Subsystem
  Right Ankle : Subsystem
  Right Hip : Subsystem
  Right Knee : Subsystem
  Right_Hip_Desired : Outport
  Right_Knee_Desired : Outport  Port=2
  Right_Ankle_Desired : Outport  Port=3
  Left_Hip_Desired : Outport  Port=4
  Left_Knee_Desired : Outport  Port=5
  Left_Ankle_Desired : Outport  Port=6
  wires:
  Offset/1 -> Left Hip/3(Offset), Right Hip/3(Offset)
  Left Knee/1(Left_Knee_Desired) -> Left_Knee_Desired/1
  W/1 -> Left Ankle/2(W), Left Knee/2(W), Left Hip/2(W), Right Hip/2(W), Right Knee/1(W), Right Ankle/2(W)
  Left Ankle/1(Left_Ankle_Desired) -> Left_Ankle_Desired/1
  Right Ankle/1(Right_Ankle_Desired) -> Right_Ankle_Desired/1
  A/1 -> Right Hip/1(A), Right Knee/2(A), Left Ankle/1(A), Left Knee/1(A), Left Hip/1(A), Right Ankle/1(A)
  Left Hip/1(Left_Hip_Desired) -> Left_Hip_Desired/1
  Right Knee/1(Right_Knee_Desired) -> Right_Knee_Desired/1
  Right Hip/1(Right_Hip_Desired) -> Right_Hip_Desired/1

== system Exo_Origianl/If Action Subsystem3/Pressure filtering ==
  u : Inport
  u1 : Inport  Port=2
  u2 : Inport  Port=3
  u3 : Inport  Port=4
  Constant1 : Constant  Value=0.9
  Delay{1..3,5} (4 alike) : Delay  DelayLength=1
  MATLAB Function1 : MATLAB Function  TreatAsAtomicUnit=on
  MATLAB Function2 : MATLAB Function  TreatAsAtomicUnit=on
  MATLAB Function3 : MATLAB Function  TreatAsAtomicUnit=on
  MATLAB Function5 : MATLAB Function  TreatAsAtomicUnit=on
  y : Outport
  y1 : Outport  Port=2
  y2 : Outport  Port=3
  y3 : Outport  Port=4
  wires:
  MATLAB Function5/1(y) -> y/1, Delay5/1
  Delay5/1 -> MATLAB Function5/3(y_delay)
  Constant1/1 -> MATLAB Function5/1(alpha), MATLAB Function3/1(alpha), MATLAB Function2/1(alpha), MATLAB Function1/1(alpha)
  MATLAB Function2/1(y) -> y2/1, Delay2/1
  MATLAB Function1/1(y) -> y1/1, Delay1/1
  MATLAB Function3/1(y) -> y3/1, Delay3/1
  Delay2/1 -> MATLAB Function2/3(y_delay)
  Delay3/1 -> MATLAB Function3/3(y_delay)
  u/1 -> MATLAB Function5/2(u)
  Delay1/1 -> MATLAB Function1/3(y_delay)
  u1/1 -> MATLAB Function1/2(u)
  u2/1 -> MATLAB Function2/2(u)
  u3/1 -> MATLAB Function3/2(u)

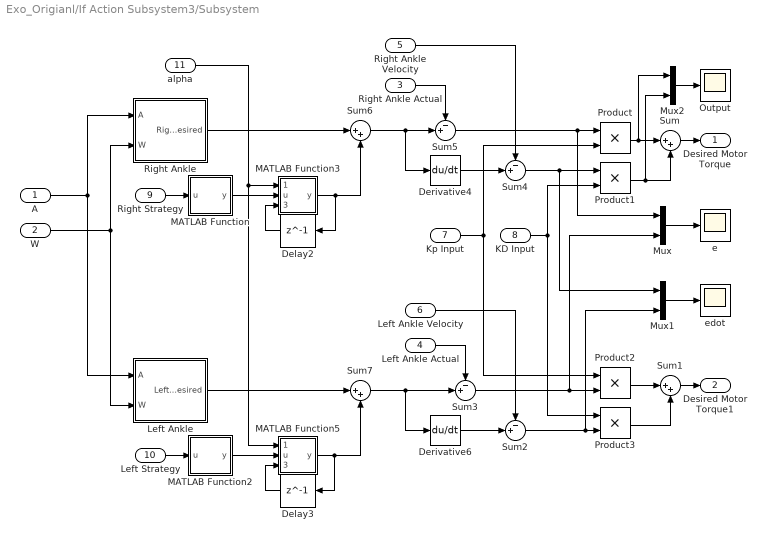
== system Exo_Origianl/If Action Subsystem3/Subsystem ==
  A : Inport
  W : Inport  Port=2
  Right Ankle Actual : Inport  Port=3
  Left Ankle Actual : Inport  Port=4
  Right Ankle Velocity : Inport  Port=5
  Left Ankle Velocity : Inport  Port=6
  Kp Input : Inport  Port=7
  KD Input : Inport  Port=8
  Right Strategy : Inport  Port=9
  Left Strategy : Inport  Port=10
  alpha : Inport  Port=11
  Delay2 : Delay  DelayLength=1
  Delay3 : Delay  DelayLength=1
  Derivative4 : Derivative
  Derivative6 : Derivative
  Left Ankle : Subsystem
  MATLAB Function : MATLAB Function  TreatAsAtomicUnit=on
  MATLAB Function2 : MATLAB Function  TreatAsAtomicUnit=on
  MATLAB Function3 : MATLAB Function  TreatAsAtomicUnit=on
  MATLAB Function5 : MATLAB Function  TreatAsAtomicUnit=on
  Mux : Mux  Inputs=2
  Mux1 : Mux  Inputs=2
  Mux2 : Mux  Inputs=2
  Output : Scope
  Product{,1..3} (4 alike) : Product
  Right Ankle : Subsystem
  Sum{,1,6..7} (4 alike) : Sum  Inputs=|++
  Sum{2..5} (4 alike) : Sum  Inputs=-+|
  e : Scope
  edot : Scope
  Desired Motor Torque : Outport
  Desired Motor Torque1 : Outport  Port=2
  wires:
  Product3/1 -> Sum1/2
  W/1 -> Right Ankle/2(W), Left Ankle/2(W)
  Product1/1 -> Mux2/2, Sum/2
  Sum3/1 -> Mux/2, Product2/2
  Sum/1 -> Desired Motor Torque/1
  Sum5/1 -> Mux/1, Product/1
  Product/1 -> Mux2/1, Sum/1
  Product2/1 -> Sum1/1
  Sum6/1 -> Derivative4/1, Sum5/2
  Sum4/1 -> Mux1/1, Product1/1
  A/1 -> Left Ankle/1(A), Right Ankle/1(A)
  Sum1/1 -> Desired Motor Torque1/1
  Sum7/1 -> Derivative6/1, Sum3/2
  Sum2/1 -> Mux1/2, Product3/2
  Mux/1 -> e/1
  Mux1/1 -> edot/1
  Right Ankle Actual/1 -> Sum5/1
  Derivative4/1 -> Sum4/2
  Right Ankle Velocity/1 -> Sum4/1
  Left Ankle Actual/1 -> Sum3/1
  Derivative6/1 -> Sum2/2
  Left Ankle Velocity/1 -> Sum2/1
  Mux2/1 -> Output/1
  KD Input/1 -> Product1/2, Product3/1
  Kp Input/1 -> Product/2, Product2/1
  Right Ankle/1(Right_Ankle_Desired) -> Sum6/1
  Right Strategy/1 -> MATLAB Function/1(u)
  Left Ankle/1(Left_Ankle_Desired) -> Sum7/1
  Left Strategy/1 -> MATLAB Function2/1(u)
  MATLAB Function/1(y) -> MATLAB Function3/2(u)
  MATLAB Function2/1(y) -> MATLAB Function5/2(u)
  Delay2/1 -> MATLAB Function3/3(y_delay)
  Delay3/1 -> MATLAB Function5/3(y_delay)
  MATLAB Function3/1(y) -> Delay2/1, Sum6/2
  alpha/1 -> MATLAB Function5/1(alpha), MATLAB Function3/1(alpha)
  MATLAB Function5/1(y) -> Delay3/1, Sum7/2

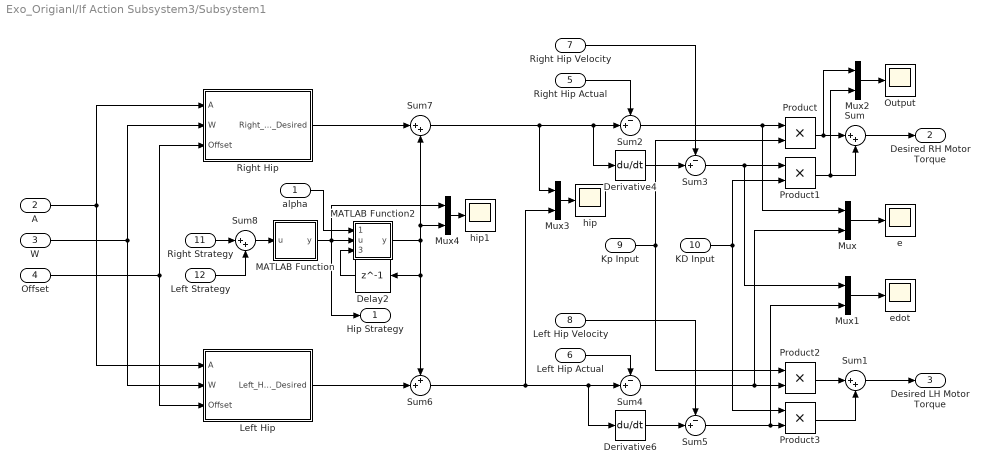
== system Exo_Origianl/If Action Subsystem3/Subsystem1 ==
  alpha : Inport
  A : Inport  Port=2
  W : Inport  Port=3
  Offset : Inport  Port=4
  Right Hip Actual : Inport  Port=5
  Left Hip Actual : Inport  Port=6
  Right Hip Velocity : Inport  Port=7
  Left Hip Velocity : Inport  Port=8
  Kp Input : Inport  Port=9
  KD Input : Inport  Port=10
  Right Strategy : Inport  Port=11
  Left Strategy : Inport  Port=12
  Delay2 : Delay  DelayLength=1
  Derivative4 : Derivative
  Derivative6 : Derivative
  Left Hip : Subsystem
  MATLAB Function : MATLAB Function  TreatAsAtomicUnit=on
  MATLAB Function2 : MATLAB Function  TreatAsAtomicUnit=on
  Mux{,1..4} (5 alike) : Mux  Inputs=2
  Output : Scope
  Product{,1..3} (4 alike) : Product
  Right Hip : Subsystem
  Sum{,1,7..8} (4 alike) : Sum  Inputs=|++
  Sum{2..5} (4 alike) : Sum  Inputs=-+|
  Sum6 : Sum  Inputs=++|
  e : Scope
  edot : Scope
  hip : Scope
  hip1 : Scope
  Hip Strategy : Outport
  Desired RH Motor Torque : Outport  Port=2
  Desired LH Motor Torque : Outport  Port=3
  wires:
  Mux2/1 -> Output/1
  Left Hip Velocity/1 -> Sum5/1
  Derivative6/1 -> Sum5/2
  Left Hip Actual/1 -> Sum4/1
  Right Hip Velocity/1 -> Sum3/1
  Derivative4/1 -> Sum3/2
  Right Hip Actual/1 -> Sum2/1
  Mux1/1 -> edot/1
  Mux/1 -> e/1
  Sum5/1 -> Product3/2, Mux1/2
  Sum6/1 -> Sum4/2, Derivative6/1, Mux3/2
  Sum1/1 -> Desired LH Motor Torque/1
  A/1 -> Right Hip/1(A), Left Hip/1(A)
  Sum3/1 -> Product1/1, Mux1/1
  Product2/1 -> Sum1/1
  Product/1 -> Sum/1, Mux2/1
  Sum2/1 -> Product/1, Mux/1
  Sum/1 -> Desired RH Motor Torque/1
  Sum4/1 -> Product2/2, Mux/2
  Product1/1 -> Sum/2, Mux2/2
  W/1 -> Right Hip/2(W), Left Hip/2(W)
  Product3/1 -> Sum1/2
  Offset/1 -> Left Hip/3(Offset), Right Hip/3(Offset)
  Kp Input/1 -> Product2/1, Product/2
  KD Input/1 -> Product3/1, Product1/2
  Right Hip/1(Right_Hip_Desired) -> Sum7/1
  Right Strategy/1 -> Sum8/1
  Left Strategy/1 -> Sum8/2
  Left Hip/1(Left_Hip_Desired) -> Sum6/2
  Sum8/1 -> MATLAB Function/1(u)
  alpha/1 -> MATLAB Function2/1(alpha)
  Mux3/1 -> hip/1
  Sum7/1 -> Mux3/1, Derivative4/1, Sum2/2
  MATLAB Function/1(y) -> Mux4/1, MATLAB Function2/2(u), Hip Strategy/1
  Mux4/1 -> hip1/1
  Delay2/1 -> MATLAB Function2/3(y_delay)
  MATLAB Function2/1(y) -> Mux4/2, Sum7/2, Sum6/1, Delay2/1

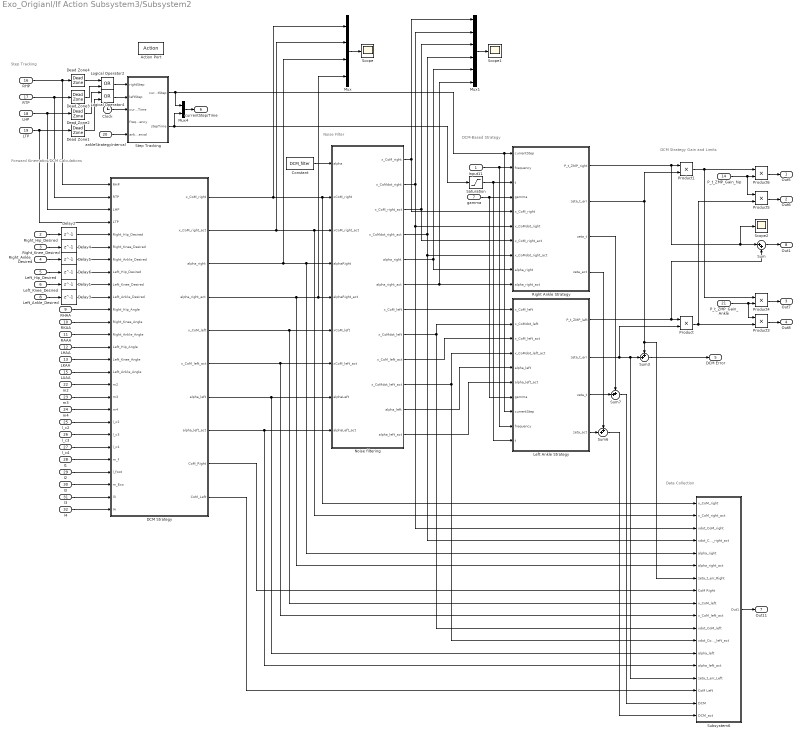
== system Exo_Origianl/If Action Subsystem3/Subsystem2 ==
  note: Noise Filter
  note: DCM-Based Strategy
  note: Data Collection
  note: Forward Kinematics/DCM Calculations
  note: Step Tracking
  note: DCM Strategy Gain and Limits
  Input11 : Inport
  Right_Hip_Desired : Inport  Port=2
  Right_Knee_Desired : Inport  Port=3
  Right_Ankle_Desired : Inport  Port=4
  Left_Hip_Desired : Inport  Port=5
  Left_Knee_Desired : Inport  Port=6
  gamma : Inport  Port=7
  Left_Ankle_Desired : Inport  Port=8
  RHAA : Inport  Port=9
  RKAA : Inport  Port=10
  RAAA : Inport  Port=11
  LHAA : Inport  Port=12
  LKAA : Inport  Port=13
  P_t_ZMP_Gain_hip : Inport  Port=14
  LAAA : Inport  Port=15
  RHP : Inport  Port=16
  RTP : Inport  Port=17
  LHP : Inport  Port=18
  LTP : Inport  Port=19
  ankleStrategyInterval : Inport  Port=20
  P_t_ZMP_Gain_Ankle : Inport  Port=21
  m2 : Inport  Port=22
  m3 : Inport  Port=23
  m4 : Inport  Port=24
  l_c2 : Inport  Port=25
  l_c3 : Inport  Port=26
  l_c4 : Inport  Port=27
  I1 : Inport  Port=28
  I2 : Inport  Port=29
  I3 : Inport  Port=30
  l3 : Inport  Port=31
  l4 : Inport  Port=32
  Action Port : ActionPort  ActionPortLabel=if(u1 > 0)
  Clock : Clock
  Constant : Constant  Value=DCM_filter
  DCM Strategy : MATLAB Function  TreatAsAtomicUnit=on
  Dead Zone{1..4} (4 alike) : DeadZone  LowerValue=0  UpperValue=pressureDeadZone
  Delay{1..6} (6 alike) : Delay  DelayLength=1
  Left Ankle Strategy : MATLAB Function  TreatAsAtomicUnit=on
  Logical Operator2 : Logic  Operator=OR  AllPortsSameDT=off  OutDataTypeStr=boolean
  Logical Operator4 : Logic  Operator=OR  AllPortsSameDT=off  OutDataTypeStr=boolean
  Mux : Mux
  Mux1 : Mux  Inputs=6
  Mux4 : Mux  Inputs=2
  Noise filtering : Subsystem
  Product{,1,3..6} (6 alike) : Product
  Right Ankle Strategy : MATLAB Function  TreatAsAtomicUnit=on
  Saturation : Saturate  UpperLimit=1.5*pi/frequency  LowerLimit=0
  Scope : Scope
  Scope1 : Scope
  Scope2 : Scope
  Step Tracking : MATLAB Function  TreatAsAtomicUnit=on
  Subsystem6 : Subsystem
  Sum : Sum  Inputs=|++
  Sum3 : Sum  Inputs=++|
  Sum6 : Sum  Inputs=++|
  Sum7 : Sum  Inputs=++|
  Out5 : Outport
  Out6 : Outport  Port=2
  Out7 : Outport  Port=3
  Out8 : Outport  Port=4
  DCM Error : Outport  Port=5
  currentStep/Time : Outport  Port=6
  Out11 : Outport  Port=7
  Out1 : Outport  Port=8
  wires:
  Product/1 -> Product5/2, Product3/2
  Product4/1 -> Out7/1
  Product1/1 -> Product6/1, Product4/1
  Mux4/1 -> currentStep/Time/1
  Product5/1 -> Out6/1
  Subsystem6/1(Out1) -> Out11/1
  Sum3/1 -> DCM Error/1
  P_t_ZMP_Gain_Ankle/1 -> Product3/1, Product4/2
  Product3/1 -> Out8/1
  Product6/1 -> Out5/1
  P_t_ZMP_Gain_hip/1 -> Product5/1, Product6/2
  Saturation/1 -> Right Ankle Strategy/3(t), Left Ankle Strategy/10(t)
  Noise filtering/1(x_CoM_right) -> Right Ankle Strategy/5(x_CoM_right), Mux1/1
  Noise filtering/11(alpha_left) -> Left Ankle Strategy/5(alpha_left)
  Noise filtering/7(x_CoM_left) -> Left Ankle Strategy/1(x_CoM_left)
  DCM Strategy/6(x_CoM_left_act) -> Noise filtering/7(xCoM_left_act), Subsystem6/10(x_CoM_left_act)
  Left Ankle Strategy/4(zeta_act) -> Sum6/2
  Right Ankle Strategy/3(zeta_t) -> Sum7/1
  Constant/1 -> Noise filtering/1(alpha)
  Noise filtering/12(alpha_left_act) -> Left Ankle Strategy/6(alpha_left_act)
  DCM Strategy/3(alpha_right) -> Mux/3, Noise filtering/4(alphaRight), Subsystem6/5(alpha_right)
  Noise filtering/4(x_CoMdot_right_act) -> Subsystem6/4(xdot_CoM_right_act), Right Ankle Strategy/8(x_CoMdot_right_act), Mux1/4
  Left Ankle Strategy/3(zeta_t) -> Sum7/2
  Noise filtering/5(alpha_right) -> Right Ankle Strategy/9(alpha_right), Mux1/5
  Step Tracking/1(currentStep) -> Right Ankle Strategy/1(currentStep), Left Ankle Strategy/8(currentStep), Mux4/1
  DCM Strategy/8(alpha_left_act) -> Noise filtering/9(alphaLeft_act), Subsystem6/14(alpha_left_act)
  DCM Strategy/4(alpha_right_act) -> Mux/4, Noise filtering/5(alphaRight_act), Subsystem6/6(alpha_right_act)
  Noise filtering/2(x_CoMdot_right) -> Right Ankle Strategy/6(x_CoMdot_right), Subsystem6/3(xdot_CoM_right), Mux1/2
  Right Ankle Strategy/4(zeta_act) -> Sum6/1
  Left Ankle Strategy/2(zeta_t_err) -> Product/2, Subsystem6/15(zeta_t_err_Left), Sum3/2
  Noise filtering/6(alpha_right_act) -> Right Ankle Strategy/10(alpha_right_act), Mux1/6
  Step Tracking/2(stepTime) -> Saturation/1, Mux4/2
  Right Ankle Strategy/2(zeta_t_err) -> Product1/2, Subsystem6/7(zeta_t_err_Right), Sum3/1
  DCM Strategy/5(x_CoM_left) -> Noise filtering/6(xCoM_left), Subsystem6/9(x_CoM_left)
  DCM Strategy/10(CoM_Left) -> Subsystem6/16(CoM Left)
  gamma/1 -> Right Ankle Strategy/4(gamma), Left Ankle Strategy/7(gamma)
  DCM Strategy/7(alpha_left) -> Subsystem6/13(alpha_left), Noise filtering/8(alphaLeft)
  DCM Strategy/2(x_CoM_right_act) -> Mux/2, Noise filtering/3(xCoM_right_act), Subsystem6/2(x_CoM_right_act)
  Noise filtering/10(x_CoMdot_left_act) -> Left Ankle Strategy/4(x_CoMdot_left_act), Subsystem6/12(xdot_CoM_left_act)
  DCM Strategy/9(CoM_Right) -> Subsystem6/8(CoM Right)
  Noise filtering/3(x_CoM_right_act) -> Right Ankle Strategy/7(x_CoM_right_act), Mux1/3
  Sum7/1 -> Subsystem6/17(DCM)
  Noise filtering/9(x_CoM_left_act) -> Left Ankle Strategy/3(x_CoM_left_act)
  Sum6/1 -> Subsystem6/18(DCM_act)
  Noise filtering/8(x_CoMdot_left) -> Subsystem6/11(xdot_CoM_left), Left Ankle Strategy/2(x_CoMdot_left)
  Dead Zone1/1 -> Logical Operator4/2
  Dead Zone4/1 -> Logical Operator2/1
  Logical Operator4/1 -> Step Tracking/2(leftStep)
  LHP/1 -> Dead Zone2/1, DCM Strategy/3(LHP)
  RHP/1 -> DCM Strategy/1(RHP), Dead Zone4/1
  LTP/1 -> Dead Zone1/1, DCM Strategy/4(LTP)
  Clock/1 -> Step Tracking/3(currentTime)
  RTP/1 -> Dead Zone3/1, DCM Strategy/2(RTP)
  Logical Operator2/1 -> Step Tracking/1(rightStep)
  Dead Zone3/1 -> Logical Operator2/2
  Dead Zone2/1 -> Logical Operator4/1
  ankleStrategyInterval/1 -> Step Tracking/5(ankleStrategyInterval)
  l3/1 -> DCM Strategy/26(l3)
  l4/1 -> DCM Strategy/27(l4)
  I3/1 -> DCM Strategy/25(m_Exo)
  I2/1 -> DCM Strategy/24(l_foot)
  I1/1 -> DCM Strategy/23(m_f)
  l_c4/1 -> DCM Strategy/22(l_c4)
  l_c3/1 -> DCM Strategy/21(l_c3)
  m3/1 -> DCM Strategy/18(m3)
  m2/1 -> DCM Strategy/17(m2)
  m4/1 -> DCM Strategy/19(m4)
  l_c2/1 -> DCM Strategy/20(l_c2)
  LAAA/1 -> DCM Strategy/16(Left_Ankle_Angle)
  LHAA/1 -> DCM Strategy/14(Left_Hip_Angle)
  LKAA/1 -> DCM Strategy/15(Left_Knee_Angle)
  RAAA/1 -> DCM Strategy/13(Right_Ankle_Angle)
  RKAA/1 -> DCM Strategy/12(Right_Knee_Angle)
  RHAA/1 -> DCM Strategy/11(Right_Hip_Angle)
  Input11/1 -> Right Ankle Strategy/2(frequency), Left Ankle Strategy/9(frequency)
  Left_Hip_Desired/1 -> Delay6/1
  Right_Knee_Desired/1 -> Delay4/1
  Right_Ankle_Desired/1 -> Delay5/1
  Left_Knee_Desired/1 -> Delay1/1
  Right_Hip_Desired/1 -> Delay2/1
  Left_Ankle_Desired/1 -> Delay3/1
  Delay1/1 -> DCM Strategy/9(Left_Knee_Desired)
  Delay5/1 -> DCM Strategy/7(Right_Ankle_Desired)
  Delay2/1 -> DCM Strategy/5(Right_Hip_Desired)
  Delay3/1 -> DCM Strategy/10(Left_Ankle_Desired)
  Delay4/1 -> DCM Strategy/6(Right_Knee_Desired)
  Delay6/1 -> DCM Strategy/8(Left_Hip_Desired)
  Mux/1 -> Scope/1
  DCM Strategy/1(x_CoM_right) -> Mux/1, Noise filtering/2(xCoM_right), Subsystem6/1(x_CoM_right)
  Mux1/1 -> Scope1/1
  Left Ankle Strategy/1(P_t_ZMP_left) -> Sum/2, Product/1
  Right Ankle Strategy/1(P_t_ZMP_right) -> Scope2/1, Sum/1, Product1/1
  Sum/1 -> Out1/1
